simulink model "Voltage_Sensor"  (R2026a)
settings: Solver=VariableStepAuto  StopTime=300
undefined symbols (not defined in the file): Sensors
settings Model: Creator=tastytaco  LastModifiedBy=tastytaco

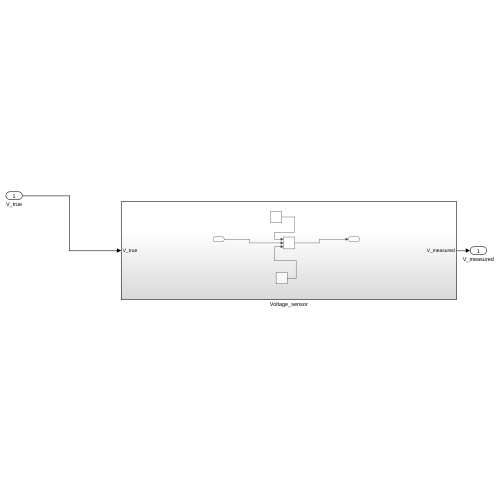
[thumbnail: Simulink's stored preview of the top-level diagram]
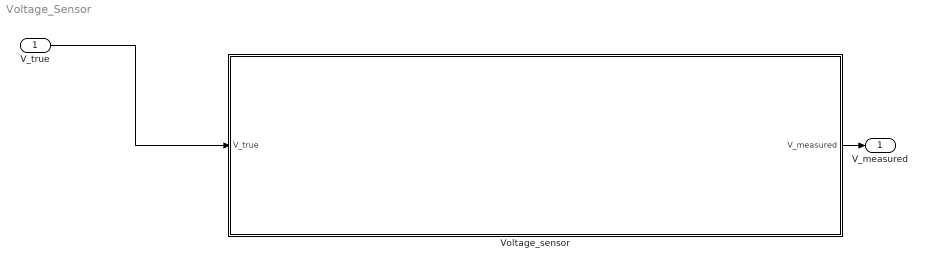
== system Voltage_Sensor ==
  V_true : Inport
  Voltage_sensor : Subsystem
  V_measured : Outport
  wires:
  Voltage_sensor/1(V_measured) -> V_measured/1
  V_true/1 -> Voltage_sensor/1(V_true)

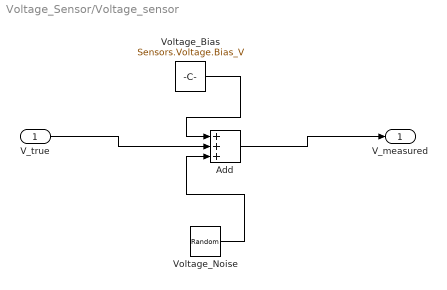
== system Voltage_Sensor/Voltage_sensor ==
  V_true : Inport
  Add : Sum  Inputs=+++
  Voltage_Bias : Constant  Value=Sensors.Voltage.Bias_V
  Voltage_Noise : RandomNumber  Mean=Sensors.Voltage.Noise_Mean_V  Variance=Sensors.Voltage.Noise_Variance_V2  Seed=12345  SampleTime=Sensors.Voltage.SampleTime
  V_measured : Outport
  wires:
  V_true/1 -> Add/2
  Voltage_Bias/1 -> Add/1
  Voltage_Noise/1 -> Add/3
  Add/1 -> V_measured/1
